simulink model "gg_plus_lc_platoon"  (R2019a)
settings: Solver=ode23t  StartTime=0.0  StopTime=70  FixedStep=0.1  MaxStep=0.01  RelTol=1e-3
InitFcn:
  | load vehStatesBus
libraries: simulink x120, powerlib_meascontrol x14, dspsigops x7, autolibshared x7
(part 4 of 7)

== system gg_plus_lc_platoon/Lo/Virtual Vehicle Following ==
  ego : Inport
  virtualLeader : Inport  Port=2
  leaderChange : Inport  Port=3
  extraSpaceFlag : Inport  Port=4
  Enable : EnablePort
  Bus Selector : BusSelector  OutputSignals=X,Xdot,u
  Bus Selector1 : BusSelector  OutputSignals=X,Xdot
  Chart : Stateflow chart  BlockKeywords=__PRM__SERIALIZED__DATA__:Stateflow Chart,Stateflow Diagram  TreatAsAtomicUnit=on
  Compare To Constant : simulink/Logic and Bit Operations/Compare To Constant  relop=>  const=0  OutDataTypeStr=boolean
  Compare To Constant1 : simulink/Logic and Bit Operations/Compare To Constant  relop=<  const=2*maxHeadwayError  OutDataTypeStr=boolean
  Compute Errors : Subsystem
  Mux : Mux  Inputs=2
  Scope : Scope  NumInputPorts=2
  Scope1 : Scope
  Sum : Sum  Inputs=-+|
  Sum6 : Sum  Inputs=|+-
  Terminator : Terminator
  Velocity Control Free Flow : Subsystem  TreatAsAtomicUnit=on
  Velocity Control Min : Subsystem  TreatAsAtomicUnit=on
  Virtual Leader Following : Subsystem  TreatAsAtomicUnit=on
  freeFlowVel : Constant  Value=freeFlowVel
  vMin : Constant  Value=vMin
  u : Outport  InitialOutput=0
  virtualErrors : Outport  Port=2  OutputWhenDisabled=reset  InitialOutput=[0, 0]
  virtualGap : Outport  Port=3  OutputWhenDisabled=reset  InitialOutput=[0]
  vLeaderInRange : Outport  Port=4
  wires:
  leaderChange/1 -> Virtual Leader Following/4(intReset), Compute Errors/6(velFilterReset)
  Compare To Constant1/1 -> Velocity Control Free Flow/3(intReset), vLeaderInRange/1, Chart/2(leaderWithinRange)
  Compare To Constant/1 -> Velocity Control Min/2(intReset)
  Velocity Control Free Flow/1(u) -> Chart/1(uFreeFlowVelControl)
  Sum/1 -> Velocity Control Min/1(ev), Chart/4(velDiff), Compare To Constant/1
  freeFlowVel/1 -> Sum6/1
  Chart/2(u) -> u/1, Scope/2
  Sum6/1 -> Velocity Control Free Flow/1(ev)
  virtualLeader/1 -> Bus Selector1/1
  Mux/1 -> virtualErrors/1
  vMin/1 -> Sum/2
  Compute Errors/1(eh) -> Compare To Constant1/1, Scope1/1, Virtual Leader Following/1(eh), Mux/1
  Bus Selector/3 -> Velocity Control Free Flow/2(realInput), Virtual Leader Following/3(realInput)  "<u>"
  ego/1 -> Bus Selector/1
  Virtual Leader Following/1(u) -> Chart/3(uVehFoll)  "uVehFoll"
  Bus Selector/2 -> Sum6/2, Sum/1, Compute Errors/2(vf)  "<Xdot>"
  Bus Selector/1 -> Compute Errors/1(xf)  "<X>"
  Compute Errors/3("gap ") -> virtualGap/1
  Compute Errors/4(unsafeFlag) -> Terminator/1
  Chart/1(state) -> Scope/1
  Bus Selector1/1 -> Compute Errors/3(xl)  "<X>"
  Velocity Control Min/1(u) -> Chart/5(uMinVelControl)  "uMinVelControl"
  Compute Errors/2(ev) -> Virtual Leader Following/2(ev), Mux/2
  extraSpaceFlag/1 -> Compute Errors/5(extraSpace)
  Bus Selector1/2 -> Compute Errors/4(vl)  "<Xdot>"

== system gg_plus_lc_platoon/Lo/controlChoice ==
  state : Inport
  follControl : Inport  Port=2
  leaderInRange : Inport  Port=3
  virtualFollControl : Inport  Port=4
  vLeaderInRange : Inport  Port=5
  ControlChoice : Stateflow chart  BlockKeywords=__PRM__SERIALIZED__DATA__:Stateflow Chart,Stateflow Diagram  TreatAsAtomicUnit=on
  Scope : Scope  NumInputPorts=2
  Scope1 : Scope  NumInputPorts=2
  u : Outport
  wires:
  state/1 -> Scope1/1, ControlChoice/1(state)
  leaderInRange/1 -> Scope1/2, ControlChoice/2(leaderInRange)
  virtualFollControl/1 -> Scope/2, ControlChoice/4(longAdjustmentData)
  follControl/1 -> Scope/1, ControlChoice/3(regVehFollData)
  ControlChoice/1(data) -> u/1  "u"
  vLeaderInRange/1 -> ControlChoice/5(vLeaderInRange)

== system gg_plus_lc_platoon/Lo/findLeader ==
  ego : Inport
  all : Inport  Port=2
  lcFlag : Inport  Port=3
  state : Inport  Port=4
  Compare To Constant : simulink/Logic and Bit Operations/Compare To Constant  relop=~=  const=4  OutDataTypeStr=boolean
  NOT : Logic  Operator=NOT  IconShape=distinctive  AllPortsSameDT=off  OutDataTypeStr=boolean
  OR : Logic  Operator=OR  IconShape=distinctive  AllPortsSameDT=off  OutDataTypeStr=boolean
  Selector : Selector  InputPortWidth=8  IndexOptions=Index vector (port)  Indices=[1]  OutputSizes=1
  Subsystem : Subsystem
  Vector Concatenate : Concatenate
  farAwayVeh : Subsystem
  leader : Outport
  leaderIdx : Outport  Port=2  InitialOutput=1
  wires:
  Vector Concatenate/1 -> Selector/1
  farAwayVeh/1(Out1) -> Vector Concatenate/2
  Selector/1 -> leader/1
  NOT/1 -> OR/1
  lcFlag/1 -> NOT/1
  OR/1 -> Subsystem/Enable
  Subsystem/1(idx) -> leaderIdx/1, Selector/2
  all/1 -> Subsystem/2(all), Vector Concatenate/1
  ego/1 -> Subsystem/1(ego), farAwayVeh/1(ego)
  state/1 -> Compare To Constant/1
  Compare To Constant/1 -> OR/2

== system gg_plus_lc_platoon/Lo/followerErrors ==
  ego : Inport
  follower : Inport  Port=2
  Bus Selector1 : BusSelector  OutputSignals=X,Xdot
  Bus Selector3 : BusSelector  OutputSignals=X,Xdot
  Mux : Mux  Inputs=2
  Sum3 : Sum  Inputs=-+|
  Terminator1 : Terminator
  gapToFollower : Subsystem
  errors : Outport
  wires:
  gapToFollower/2("gap ") -> Terminator1/1
  Sum3/1 -> Mux/2
  Bus Selector3/2 -> gapToFollower/2(vf), Sum3/1  "<Xdot>"
  follower/1 -> Bus Selector3/1
  gapToFollower/1(eh) -> Mux/1
  Bus Selector1/2 -> Sum3/2  "<Xdot>"
  Bus Selector3/1 -> gapToFollower/1(xf)  "<X>"
  ego/1 -> Bus Selector1/1
  Bus Selector1/1 -> gapToFollower/3(xl)  "<X>"
  Mux/1 -> errors/1

== system gg_plus_lc_platoon/Lo/maneuverState ==
  note: States are:
      | 0 - Lane keeping
      | 1 - Longitudinal Adjustment
      | 2 - Steady State
      | 3 - Safe to LC
      | 4 - Performing LC
      | 5 - LC is done
  longAdj : Inport
  steadyState : Inport  Port=2
  safeToVirtualFoll : Inport  Port=3
  canStartLC : Inport  Port=4
  lcDone : Inport  Port=5
  Enable : EnablePort
  AND{,1..3} (4 alike) : Logic  IconShape=distinctive  AllPortsSameDT=off  OutDataTypeStr=fixdt(1,16)
  Data Type Conversion : DataTypeConversion  OutMin=0  OutMax=1  OutDataTypeStr=fixdt(1,16)
  Scope : Scope  NumInputPorts=5
  Sum : Sum  Inputs=+++++
  state : Outport  InitialOutput=0
  wires:
  AND3/1 -> Scope/5, Sum/5
  AND2/1 -> AND3/1, Scope/4, Sum/4
  AND1/1 -> AND2/1, Scope/3, Sum/3
  AND/1 -> AND1/1, Scope/2, Sum/2
  Sum/1 -> state/1
  lcDone/1 -> AND3/2
  canStartLC/1 -> AND2/2
  safeToVirtualFoll/1 -> AND1/2
  steadyState/1 -> AND/2
  longAdj/1 -> Data Type Conversion/1, AND/1
  Data Type Conversion/1 -> Scope/1, Sum/1

== system gg_plus_lc_platoon/Lo/safeErrors ==
  errors : Inport
  AND : Logic  IconShape=distinctive  AllPortsSameDT=off  OutDataTypeStr=boolean
  Compare To Constant4 : simulink/Logic and Bit Operations/Compare To Constant  relop=>=  const=-0.1  OutDataTypeStr=boolean
  Demux : Demux  Outputs=2
  Demux1 : Demux  Outputs=2
  Memory : Memory
  Scope : Scope  NumInputPorts=2
  Triggered Subsystem1 : Subsystem  TreatAsAtomicUnit=on
  safetyFlag : Outport
  wires:
  Demux1/2 -> Scope/2
  Demux1/1 -> Scope/1
  Demux/2 -> AND/2
  Demux/1 -> AND/1
  AND/1 -> Triggered Subsystem1/Trigger
  errors/1 -> Compare To Constant4/1, Demux1/1
  Compare To Constant4/1 -> Demux/1
  Triggered Subsystem1/1(Out1) -> Memory/1
  Memory/1 -> safetyFlag/1

== system gg_plus_lc_platoon/Lo/virtualVehiclesManager ==
  all : Inport
  longAdj : Inport  Port=2
  lcFlag : Inport  Port=3
  lcDone : Inport  Port=4
  posInPlatoon : Inport  Port=5
  lcStrategy : Inport  Port=6
  Detect Change : simulink/Logic and Bit Operations/Detect Change  vinit=0  OutDataTypeStr=boolean
  MATLAB Function : MATLAB Function  TreatAsAtomicUnit=on
  MATLAB Function1 : MATLAB Function  TreatAsAtomicUnit=on
  Selector : Selector  InputPortWidth=7  IndexOptions=Index vector (port)  Indices=[1]  OutputSizes=1
  Selector1 : Selector  InputPortWidth=7  IndexOptions=Index vector (port)  Indices=[1]  OutputSizes=1
  Width : Width
  virtualVehs : Scope  NumInputPorts=2
  virtualLeader : Outport
  leaderChange : Outport  Port=2
  virtualFollower : Outport  Port=3
  wires:
  Detect Change/1 -> leaderChange/1
  Selector/1 -> virtualLeader/1
  all/1 -> Width/1, Selector1/1, Selector/1
  lcStrategy/1 -> MATLAB Function1/5(lcStrategy), MATLAB Function/6(lcStrategy)
  posInPlatoon/1 -> MATLAB Function1/4(posInPlatoon), MATLAB Function/5(posInPlatoon)
  lcFlag/1 -> MATLAB Function1/3(lcFlag), MATLAB Function/3(lcFlag)
  Width/1 -> MATLAB Function1/1(nVehicles), MATLAB Function/1(nVehicles)
  lcDone/1 -> MATLAB Function/4(lcDone)
  Selector1/1 -> virtualFollower/1
  longAdj/1 -> MATLAB Function1/2(longAdj), MATLAB Function/2(longAdj)
  MATLAB Function/1(virtualLeaderIdx) -> virtualVehs/1, Detect Change/1, Selector/2
  MATLAB Function1/1(virtualFollowerIdx) -> Selector1/2, virtualVehs/2

== system gg_plus_lc_platoon/p1/Lateral Control ==
  <Y> : Inport
  <r> : Inport  Port=2
  startLaneChange : Inport  Port=3
  yRef : Inport  Port=4
  Demux2 : Demux
  Full State Observer : Subsystem
  Gain1 : Gain  Gain=Klat  Multiplication=Matrix(K*u)
  Integrator : Integrator  InitialCondition=y0
  Mux : Mux  Inputs=2
  Pad : dspsigops/Pad  padAlong=Columns  dimsToPad=1  valSrc=Specify via dialog  padVal=0  spec=Output size  padNumOutRowsSpecMethod=User-specified  numOutRows=4  padNumOutColsSpecMethod=User-specified  numOutCols=1  isVarDimsMode=off  padBeginning=0  padEnd=0  outSizeMode=User-specified  outSize=1  padSigAt=End  trunc_flag=None  roundingMode=Floor  overflowMode=off  truncOrWrapMode=Truncate  wrap_flag=None
      settings: SourceProductName=DSP System Toolbox  SourceProductBaseCode=DS
  Rate Limiter : RateLimiter  RisingSlewLimit=maxDeltaDot  FallingSlewLimit=-maxDeltaDot  SampleTimeMode=inherited
  Saturation : Saturate  UpperLimit=maxDelta  LowerLimit=-maxDelta
  Scope : Scope  NumInputPorts=4
  Scope1 : Scope
  Sum : Sum  Inputs=|+-
  Sum2 : Sum  Inputs=|+-
  Triggered Subsystem1 : Subsystem  TreatAsAtomicUnit=on
  delta : Outport
  wires:
  yRef/1 -> Triggered Subsystem1/1(In1)
  startLaneChange/1 -> Triggered Subsystem1/Trigger
  <Y>/1 -> Mux/1
  Triggered Subsystem1/1(Out1) -> Sum2/1
  Demux2/3 -> Scope/3
  Saturation/1 -> Rate Limiter/1
  Sum2/1 -> Integrator/1
  Demux2/2 -> Scope/2
  Demux2/4 -> Scope/4
  Mux/1 -> Full State Observer/1(measuredOutputs)
  Pad/1 -> Sum/1
  Sum/1 -> Gain1/1
  Full State Observer/1(xhat) -> Demux2/1, Sum/2  "estStates"
  <r>/1 -> Mux/2
  Gain1/1 -> Saturation/1
  Integrator/1 -> Pad/1, Sum2/2
  Demux2/1 -> Scope/1
  Rate Limiter/1 -> delta/1, Scope1/1, Full State Observer/2(delta)  "delta"

== system gg_plus_lc_platoon/p1/Regular Vehicle Following ==
  ego : Inport
  leader : Inport  Port=2
  leaderChange : Inport  Port=3
  extraSpaceFlag : Inport  Port=4
  Bus Selector : BusSelector  OutputSignals=X,Xdot,u
  Bus Selector1 : BusSelector  OutputSignals=X,Xdot
  Compare To Constant : simulink/Logic and Bit Operations/Compare To Constant  relop=<  const=5*maxHeadwayError  OutDataTypeStr=boolean
  Compute Errors : Subsystem
  Constant : Constant  Value=0
  Mux : Mux  Inputs=2
  Rate Limiter : RateLimiter  RisingSlewLimit=maxJerk  FallingSlewLimit=minJerk  SampleTimeMode=inherited
  Rate Limiter1 : RateLimiter  RisingSlewLimit=maxComfJerk  FallingSlewLimit=minComfJerk  SampleTimeMode=inherited
  Scope : Scope
  Scope2 : Scope
  Switch : Switch  Criteria=u2 > Threshold
  Switch1 : Switch  Criteria=u2 > Threshold
  Veh Following : Subsystem  TreatAsAtomicUnit=on
  Velocity Control : Subsystem  TreatAsAtomicUnit=on
  XOR : Logic  Operator=XOR  IconShape=distinctive  AllPortsSameDT=off  OutDataTypeStr=boolean
  comf saturation : Saturate  UpperLimit=maxComfAccel  LowerLimit=minComfAccel
  eh : Scope
  output : Scope
  safe saturation : Saturate  UpperLimit=maxAcceleration  LowerLimit=minAcceleration
  veh foll state : Scope  NumInputPorts=2
  u : Outport
  errors : Outport  Port=2
  gap : Outport  Port=3
  leaderInRange : Outport  Port=4
  wires:
  Constant/1 -> Compute Errors/6(velFilterReset)
  XOR/1 -> Veh Following/4(intReset)
  Bus Selector1/2 -> Compute Errors/4(vl)  "<Xdot>"
  leader/1 -> Bus Selector1/1
  Compare To Constant/1 -> Velocity Control/3(intReset), XOR/2, leaderInRange/1, veh foll state/1, Switch/2
  Mux/1 -> errors/1
  Bus Selector1/1 -> Compute Errors/3(xl)  "<X>"
  Velocity Control/1(u) -> Switch/3
  Compute Errors/2(ev) -> Veh Following/2(ev), Mux/2
  comf saturation/1 -> Rate Limiter1/1
  safe saturation/1 -> Rate Limiter/1
  Rate Limiter/1 -> Switch1/1  "sat(u)"
  Switch1/1 -> output/1, u/1
  Switch/1 -> comf saturation/1, veh foll state/2, safe saturation/1
  Bus Selector/3 -> Velocity Control/2(realInput), Veh Following/3(realInput)  "<u>"
  Rate Limiter1/1 -> Switch1/3  "sat(u)"
  Compute Errors/4(unsafeFlag) -> Scope2/1, Switch1/2
  Compute Errors/3("gap ") -> gap/1
  ego/1 -> Bus Selector/1
  Compute Errors/1(eh) -> Mux/1, Veh Following/1(eh), Scope/1, Compare To Constant/1, eh/1
  extraSpaceFlag/1 -> Compute Errors/5(extraSpaceFlag)
  Veh Following/1(u) -> Switch/1
  Bus Selector/1 -> Compute Errors/1(xf)  "<X>"
  Bus Selector/2 -> Compute Errors/2(vf), Velocity Control/1(velocity)  "<Xdot>"
  leaderChange/1 -> XOR/1

== system gg_plus_lc_platoon/p1/Subsystem ==
  u : Inport
  state : Inport  Port=2
  Compare To Constant : simulink/Logic and Bit Operations/Compare To Constant  relop===  const=4  OutDataTypeStr=boolean
  Scope : Scope
  Switch1 : Switch  Criteria=u2 > Threshold
  comf saturation : Saturate  UpperLimit=maxComfAccel  LowerLimit=minComfAccel
  comf jerk : RateLimiter  RisingSlewLimit=maxComfJerk  FallingSlewLimit=minComfJerk  SampleTimeMode=inherited
  safe saturation : Saturate  UpperLimit=maxAcceleration  LowerLimit=minAcceleration
  safe jerk : RateLimiter  RisingSlewLimit=maxJerk  FallingSlewLimit=minJerk  SampleTimeMode=inherited
  sat(u) : Outport
  wires:
  safe saturation/1 -> safe jerk/1
  safe jerk/1 -> Switch1/1
  comf saturation/1 -> comf jerk/1
  state/1 -> Compare To Constant/1
  u/1 -> comf saturation/1, safe saturation/1
  comf jerk/1 -> Switch1/3
  Switch1/1 -> Scope/1, sat(u)/1
  Compare To Constant/1 -> Switch1/2

== system gg_plus_lc_platoon/p1/Subsystem1 ==
  u : Inport
  errors : Inport  Port=2
  virtualErrors : Inport  Port=3
  extraSpaceFlag : Inport  Port=4
  AND1 : Logic  Inputs=4  IconShape=distinctive  AllPortsSameDT=off  OutDataTypeStr=boolean
  Memory : Memory
  Triggered Subsystem1 : Subsystem  TreatAsAtomicUnit=on
  safeErrors1 : Subsystem
  safeErrors2 : Subsystem
  steadyState : Subsystem
  longAdjDone : Outport
  wires:
  u/1 -> steadyState/1(u)
  safeErrors1/1(safetyFlag) -> AND1/2
  steadyState/1(ssFlag) -> AND1/1
  extraSpaceFlag/1 -> AND1/4
  virtualErrors/1 -> safeErrors2/1(errors)
  safeErrors2/1(safetyFlag) -> AND1/3
  AND1/1 -> Triggered Subsystem1/Trigger
  Triggered Subsystem1/1(Out1) -> Memory/1
  errors/1 -> safeErrors1/1(errors)
  Memory/1 -> longAdjDone/1

== system gg_plus_lc_platoon/p1/Subsystem2 ==
  posInPlatoon : Inport
  strategy : Inport  Port=2
  platoonState : Inport  Port=3
  Enable : EnablePort
  MATLAB Function : MATLAB Function  TreatAsAtomicUnit=on
  longAdj : Outport
  wires:
  MATLAB Function/1(longAdjFlag) -> longAdj/1
  platoonState/1 -> MATLAB Function/3(platoonState)
  posInPlatoon/1 -> MATLAB Function/2(posInPlatoon)
  strategy/1 -> MATLAB Function/1(strategy)

== system gg_plus_lc_platoon/p1/Subsystem3 ==
  strategy : Inport
  platoonStates : Inport  Port=2
  Compare To Constant : simulink/Logic and Bit Operations/Compare To Constant  relop=>  const=1  OutDataTypeStr=boolean
  Compare To Constant1 : simulink/Logic and Bit Operations/Compare To Constant  relop=>  const=2  OutDataTypeStr=boolean
  OR : Logic  Operator=OR  IconShape=distinctive  AllPortsSameDT=off  OutDataTypeStr=boolean
  Selector : Selector  IndexOptions=Index vector (port)  Indices=[1 3]  OutputSizes=1
  Width : Width
  Out1 : Outport
  wires:
  Compare To Constant1/1 -> OR/2
  Selector/1 -> Compare To Constant1/1
  Width/1 -> Selector/2
  platoonStates/1 -> Selector/1, Width/1
  OR/1 -> Out1/1
  Compare To Constant/1 -> OR/1
  strategy/1 -> Compare To Constant/1

== system gg_plus_lc_platoon/p1/Triggered Subsystem ==
  Trigger : TriggerPort  VariantControl=Variant
  Constant : Constant
  lcFlag : Outport  InitialOutput=0
  wires:
  Constant/1 -> lcFlag/1

== system gg_plus_lc_platoon/p1/Virtual Vehicle Following ==
  ego : Inport
  virtualLeader : Inport  Port=2
  leaderChange : Inport  Port=3
  extraSpaceFlag : Inport  Port=4
  Enable : EnablePort
  Bus Selector : BusSelector  OutputSignals=X,Xdot,u
  Bus Selector1 : BusSelector  OutputSignals=X,Xdot
  Chart : Stateflow chart  BlockKeywords=__PRM__SERIALIZED__DATA__:Stateflow Chart,Stateflow Diagram  TreatAsAtomicUnit=on
  Compare To Constant : simulink/Logic and Bit Operations/Compare To Constant  relop=>  const=0  OutDataTypeStr=boolean
  Compare To Constant1 : simulink/Logic and Bit Operations/Compare To Constant  relop=<  const=2*maxHeadwayError  OutDataTypeStr=boolean
  Compute Errors : Subsystem
  Mux : Mux  Inputs=2
  Scope : Scope  NumInputPorts=2
  Scope1 : Scope
  Sum : Sum  Inputs=-+|
  Sum6 : Sum  Inputs=|+-
  Terminator : Terminator
  Velocity Control Free Flow : Subsystem  TreatAsAtomicUnit=on
  Velocity Control Min : Subsystem  TreatAsAtomicUnit=on
  Virtual Leader Following : Subsystem  TreatAsAtomicUnit=on
  freeFlowVel : Constant  Value=freeFlowVel
  vMin : Constant  Value=vMin
  u : Outport  InitialOutput=0
  virtualErrors : Outport  Port=2  OutputWhenDisabled=reset  InitialOutput=[0, 0]
  virtualGap : Outport  Port=3  OutputWhenDisabled=reset  InitialOutput=[0]
  vLeaderInRange : Outport  Port=4
  wires:
  Bus Selector1/2 -> Compute Errors/4(vl)  "<Xdot>"
  extraSpaceFlag/1 -> Compute Errors/5(extraSpace)
  Compute Errors/2(ev) -> Mux/2, Virtual Leader Following/2(ev)
  Velocity Control Min/1(u) -> Chart/5(uMinVelControl)  "uMinVelControl"
  Bus Selector1/1 -> Compute Errors/3(xl)  "<X>"
  Chart/1(state) -> Scope/1
  Compute Errors/4(unsafeFlag) -> Terminator/1
  Compute Errors/3("gap ") -> virtualGap/1
  Bus Selector/1 -> Compute Errors/1(xf)  "<X>"
  Bus Selector/2 -> Compute Errors/2(vf), Sum/1, Sum6/2  "<Xdot>"
  Virtual Leader Following/1(u) -> Chart/3(uVehFoll)  "uVehFoll"
  ego/1 -> Bus Selector/1
  Bus Selector/3 -> Virtual Leader Following/3(realInput), Velocity Control Free Flow/2(realInput)  "<u>"
  Compute Errors/1(eh) -> Mux/1, Virtual Leader Following/1(eh), Scope1/1, Compare To Constant1/1
  vMin/1 -> Sum/2
  Mux/1 -> virtualErrors/1
  virtualLeader/1 -> Bus Selector1/1
  Sum6/1 -> Velocity Control Free Flow/1(ev)
  Chart/2(u) -> Scope/2, u/1
  freeFlowVel/1 -> Sum6/1
  Sum/1 -> Compare To Constant/1, Chart/4(velDiff), Velocity Control Min/1(ev)
  Velocity Control Free Flow/1(u) -> Chart/1(uFreeFlowVelControl)
  Compare To Constant/1 -> Velocity Control Min/2(intReset)
  Compare To Constant1/1 -> Chart/2(leaderWithinRange), vLeaderInRange/1, Velocity Control Free Flow/3(intReset)
  leaderChange/1 -> Compute Errors/6(velFilterReset), Virtual Leader Following/4(intReset)

== system gg_plus_lc_platoon/p1/controlChoice ==
  state : Inport
  follControl : Inport  Port=2
  leaderInRange : Inport  Port=3
  virtualFollControl : Inport  Port=4
  vLeaderInRange : Inport  Port=5
  ControlChoice : Stateflow chart  BlockKeywords=__PRM__SERIALIZED__DATA__:Stateflow Chart,Stateflow Diagram  TreatAsAtomicUnit=on
  Scope : Scope  NumInputPorts=2
  Scope1 : Scope  NumInputPorts=2
  u : Outport
  wires:
  vLeaderInRange/1 -> ControlChoice/5(vLeaderInRange)
  ControlChoice/1(data) -> u/1  "u"
  follControl/1 -> ControlChoice/3(regVehFollData), Scope/1
  virtualFollControl/1 -> ControlChoice/4(longAdjustmentData), Scope/2
  leaderInRange/1 -> ControlChoice/2(leaderInRange), Scope1/2
  state/1 -> ControlChoice/1(state), Scope1/1

== system gg_plus_lc_platoon/p1/findLeader ==
  ego : Inport
  all : Inport  Port=2
  lcFlag : Inport  Port=3
  state : Inport  Port=4
  Compare To Constant : simulink/Logic and Bit Operations/Compare To Constant  relop=~=  const=4  OutDataTypeStr=boolean
  NOT : Logic  Operator=NOT  IconShape=distinctive  AllPortsSameDT=off  OutDataTypeStr=boolean
  OR : Logic  Operator=OR  IconShape=distinctive  AllPortsSameDT=off  OutDataTypeStr=boolean
  Selector : Selector  InputPortWidth=8  IndexOptions=Index vector (port)  Indices=[1]  OutputSizes=1
  Subsystem : Subsystem
  Vector Concatenate : Concatenate
  farAwayVeh : Subsystem
  leader : Outport
  leaderIdx : Outport  Port=2  InitialOutput=1
  wires:
  Compare To Constant/1 -> OR/2
  state/1 -> Compare To Constant/1
  ego/1 -> farAwayVeh/1(ego), Subsystem/1(ego)
  all/1 -> Vector Concatenate/1, Subsystem/2(all)
  Subsystem/1(idx) -> Selector/2, leaderIdx/1
  OR/1 -> Subsystem/Enable
  lcFlag/1 -> NOT/1
  NOT/1 -> OR/1
  Selector/1 -> leader/1
  farAwayVeh/1(Out1) -> Vector Concatenate/2
  Vector Concatenate/1 -> Selector/1

== system gg_plus_lc_platoon/p1/followerErrors ==
  ego : Inport
  follower : Inport  Port=2
  Bus Selector1 : BusSelector  OutputSignals=X,Xdot
  Bus Selector3 : BusSelector  OutputSignals=X,Xdot
  Mux : Mux  Inputs=2
  Sum3 : Sum  Inputs=-+|
  Terminator1 : Terminator
  gapToFollower : Subsystem
  errors : Outport
  wires:
  Mux/1 -> errors/1
  Bus Selector1/1 -> gapToFollower/3(xl)  "<X>"
  ego/1 -> Bus Selector1/1
  Bus Selector3/1 -> gapToFollower/1(xf)  "<X>"
  Bus Selector1/2 -> Sum3/2  "<Xdot>"
  gapToFollower/1(eh) -> Mux/1
  follower/1 -> Bus Selector3/1
  Bus Selector3/2 -> Sum3/1, gapToFollower/2(vf)  "<Xdot>"
  Sum3/1 -> Mux/2
  gapToFollower/2("gap ") -> Terminator1/1

== system gg_plus_lc_platoon/p1/maneuverState ==
  note: States are:
      | 0 - Lane keeping
      | 1 - Longitudinal Adjustment
      | 2 - Steady State
      | 3 - Safe to LC
      | 4 - Performing LC
      | 5 - LC is done
  longAdj : Inport
  steadyState : Inport  Port=2
  safeToVirtualFoll : Inport  Port=3
  canStartLC : Inport  Port=4
  lcDone : Inport  Port=5
  Enable : EnablePort
  AND{,1..3} (4 alike) : Logic  IconShape=distinctive  AllPortsSameDT=off  OutDataTypeStr=fixdt(1,16)
  Data Type Conversion : DataTypeConversion  OutMin=0  OutMax=1  OutDataTypeStr=fixdt(1,16)
  Scope : Scope  NumInputPorts=5
  Sum : Sum  Inputs=+++++
  state : Outport  InitialOutput=0
  wires:
  Data Type Conversion/1 -> Sum/1, Scope/1
  longAdj/1 -> AND/1, Data Type Conversion/1
  steadyState/1 -> AND/2
  safeToVirtualFoll/1 -> AND1/2
  canStartLC/1 -> AND2/2
  lcDone/1 -> AND3/2
  Sum/1 -> state/1
  AND/1 -> Sum/2, Scope/2, AND1/1
  AND1/1 -> Sum/3, Scope/3, AND2/1
  AND2/1 -> Sum/4, Scope/4, AND3/1
  AND3/1 -> Sum/5, Scope/5

== system gg_plus_lc_platoon/p1/safeErrors ==
  errors : Inport
  AND : Logic  IconShape=distinctive  AllPortsSameDT=off  OutDataTypeStr=boolean
  Compare To Constant4 : simulink/Logic and Bit Operations/Compare To Constant  relop=>=  const=-0.1  OutDataTypeStr=boolean
  Demux : Demux  Outputs=2
  Demux1 : Demux  Outputs=2
  Memory : Memory
  Scope : Scope  NumInputPorts=2
  Triggered Subsystem1 : Subsystem  TreatAsAtomicUnit=on
  safetyFlag : Outport
  wires:
  Memory/1 -> safetyFlag/1
  Triggered Subsystem1/1(Out1) -> Memory/1
  Compare To Constant4/1 -> Demux/1
  errors/1 -> Demux1/1, Compare To Constant4/1
  AND/1 -> Triggered Subsystem1/Trigger
  Demux/1 -> AND/1
  Demux/2 -> AND/2
  Demux1/1 -> Scope/1
  Demux1/2 -> Scope/2

== system gg_plus_lc_platoon/p1/virtualVehiclesManager ==
  all : Inport
  longAdj : Inport  Port=2
  lcFlag : Inport  Port=3
  lcDone : Inport  Port=4
  posInPlatoon : Inport  Port=5
  lcStrategy : Inport  Port=6
  Detect Change : simulink/Logic and Bit Operations/Detect Change  vinit=0  OutDataTypeStr=boolean
  MATLAB Function : MATLAB Function  TreatAsAtomicUnit=on
  MATLAB Function1 : MATLAB Function  TreatAsAtomicUnit=on
  Selector : Selector  InputPortWidth=7  IndexOptions=Index vector (port)  Indices=[1]  OutputSizes=1
  Selector1 : Selector  InputPortWidth=7  IndexOptions=Index vector (port)  Indices=[1]  OutputSizes=1
  Width : Width
  virtualVehs : Scope  NumInputPorts=2
  virtualLeader : Outport
  leaderChange : Outport  Port=2
  virtualFollower : Outport  Port=3
  wires:
  MATLAB Function1/1(virtualFollowerIdx) -> virtualVehs/2, Selector1/2
  MATLAB Function/1(virtualLeaderIdx) -> Selector/2, Detect Change/1, virtualVehs/1
  longAdj/1 -> MATLAB Function/2(longAdj), MATLAB Function1/2(longAdj)
  Selector1/1 -> virtualFollower/1
  lcDone/1 -> MATLAB Function/4(lcDone)
  Width/1 -> MATLAB Function/1(nVehicles), MATLAB Function1/1(nVehicles)
  lcFlag/1 -> MATLAB Function/3(lcFlag), MATLAB Function1/3(lcFlag)
  posInPlatoon/1 -> MATLAB Function/5(posInPlatoon), MATLAB Function1/4(posInPlatoon)
  lcStrategy/1 -> MATLAB Function/6(lcStrategy), MATLAB Function1/5(lcStrategy)
  all/1 -> Selector/1, Selector1/1, Width/1
  Selector/1 -> virtualLeader/1
  Detect Change/1 -> leaderChange/1

== system gg_plus_lc_platoon/p2/Lateral Control ==
  <Y> : Inport
  <r> : Inport  Port=2
  startLaneChange : Inport  Port=3
  yRef : Inport  Port=4
  Demux2 : Demux
  Full State Observer : Subsystem
  Gain1 : Gain  Gain=Klat  Multiplication=Matrix(K*u)
  Integrator : Integrator  InitialCondition=y0
  Mux : Mux  Inputs=2
  Pad : dspsigops/Pad  padAlong=Columns  dimsToPad=1  valSrc=Specify via dialog  padVal=0  spec=Output size  padNumOutRowsSpecMethod=User-specified  numOutRows=4  padNumOutColsSpecMethod=User-specified  numOutCols=1  isVarDimsMode=off  padBeginning=0  padEnd=0  outSizeMode=User-specified  outSize=1  padSigAt=End  trunc_flag=None  roundingMode=Floor  overflowMode=off  truncOrWrapMode=Truncate  wrap_flag=None
      settings: SourceProductName=DSP System Toolbox  SourceProductBaseCode=DS
  Rate Limiter : RateLimiter  RisingSlewLimit=maxDeltaDot  FallingSlewLimit=-maxDeltaDot  SampleTimeMode=inherited
  Saturation : Saturate  UpperLimit=maxDelta  LowerLimit=-maxDelta
  Scope : Scope  NumInputPorts=4
  Scope1 : Scope
  Sum : Sum  Inputs=|+-
  Sum2 : Sum  Inputs=|+-
  Triggered Subsystem1 : Subsystem  TreatAsAtomicUnit=on
  delta : Outport
  wires:
  Rate Limiter/1 -> Full State Observer/2(delta), Scope1/1, delta/1  "delta"
  Demux2/1 -> Scope/1
  Integrator/1 -> Sum2/2, Pad/1
  Gain1/1 -> Saturation/1
  <r>/1 -> Mux/2
  Full State Observer/1(xhat) -> Sum/2, Demux2/1  "estStates"
  Sum/1 -> Gain1/1
  Pad/1 -> Sum/1
  Mux/1 -> Full State Observer/1(measuredOutputs)
  Demux2/4 -> Scope/4
  Demux2/2 -> Scope/2
  Sum2/1 -> Integrator/1
  Saturation/1 -> Rate Limiter/1
  Demux2/3 -> Scope/3
  Triggered Subsystem1/1(Out1) -> Sum2/1
  <Y>/1 -> Mux/1
  startLaneChange/1 -> Triggered Subsystem1/Trigger
  yRef/1 -> Triggered Subsystem1/1(In1)

== system gg_plus_lc_platoon/p2/Regular Vehicle Following ==
  ego : Inport
  leader : Inport  Port=2
  leaderChange : Inport  Port=3
  extraSpaceFlag : Inport  Port=4
  Bus Selector : BusSelector  OutputSignals=X,Xdot,u
  Bus Selector1 : BusSelector  OutputSignals=X,Xdot
  Compare To Constant : simulink/Logic and Bit Operations/Compare To Constant  relop=<  const=5*maxHeadwayError  OutDataTypeStr=boolean
  Compute Errors : Subsystem
  Constant : Constant  Value=0
  Mux : Mux  Inputs=2
  Rate Limiter : RateLimiter  RisingSlewLimit=maxJerk  FallingSlewLimit=minJerk  SampleTimeMode=inherited
  Rate Limiter1 : RateLimiter  RisingSlewLimit=maxComfJerk  FallingSlewLimit=minComfJerk  SampleTimeMode=inherited
  Scope : Scope
  Scope2 : Scope
  Switch : Switch  Criteria=u2 > Threshold
  Switch1 : Switch  Criteria=u2 > Threshold
  Veh Following : Subsystem  TreatAsAtomicUnit=on
  Velocity Control : Subsystem  TreatAsAtomicUnit=on
  XOR : Logic  Operator=XOR  IconShape=distinctive  AllPortsSameDT=off  OutDataTypeStr=boolean
  comf saturation : Saturate  UpperLimit=maxComfAccel  LowerLimit=minComfAccel
  eh : Scope
  output : Scope
  safe saturation : Saturate  UpperLimit=maxAcceleration  LowerLimit=minAcceleration
  veh foll state : Scope  NumInputPorts=2
  u : Outport
  errors : Outport  Port=2
  gap : Outport  Port=3
  leaderInRange : Outport  Port=4
  wires:
  leaderChange/1 -> XOR/1
  Bus Selector/2 -> Velocity Control/1(velocity), Compute Errors/2(vf)  "<Xdot>"
  Bus Selector/1 -> Compute Errors/1(xf)  "<X>"
  Veh Following/1(u) -> Switch/1
  extraSpaceFlag/1 -> Compute Errors/5(extraSpaceFlag)
  Compute Errors/1(eh) -> eh/1, Compare To Constant/1, Scope/1, Veh Following/1(eh), Mux/1
  ego/1 -> Bus Selector/1
  Compute Errors/3("gap ") -> gap/1
  Compute Errors/4(unsafeFlag) -> Switch1/2, Scope2/1
  Rate Limiter1/1 -> Switch1/3  "sat(u)"
  Bus Selector/3 -> Veh Following/3(realInput), Velocity Control/2(realInput)  "<u>"
  Switch/1 -> safe saturation/1, veh foll state/2, comf saturation/1
  Switch1/1 -> u/1, output/1
  Rate Limiter/1 -> Switch1/1  "sat(u)"
  safe saturation/1 -> Rate Limiter/1
  comf saturation/1 -> Rate Limiter1/1
  Compute Errors/2(ev) -> Mux/2, Veh Following/2(ev)
  Velocity Control/1(u) -> Switch/3
  Bus Selector1/1 -> Compute Errors/3(xl)  "<X>"
  Mux/1 -> errors/1
  Compare To Constant/1 -> Switch/2, veh foll state/1, leaderInRange/1, XOR/2, Velocity Control/3(intReset)
  leader/1 -> Bus Selector1/1
  Bus Selector1/2 -> Compute Errors/4(vl)  "<Xdot>"
  XOR/1 -> Veh Following/4(intReset)
  Constant/1 -> Compute Errors/6(velFilterReset)

== system gg_plus_lc_platoon/p2/Subsystem ==
  u : Inport
  state : Inport  Port=2
  Compare To Constant : simulink/Logic and Bit Operations/Compare To Constant  relop===  const=4  OutDataTypeStr=boolean
  Scope : Scope
  Switch1 : Switch  Criteria=u2 > Threshold
  comf saturation : Saturate  UpperLimit=maxComfAccel  LowerLimit=minComfAccel
  comf jerk : RateLimiter  RisingSlewLimit=maxComfJerk  FallingSlewLimit=minComfJerk  SampleTimeMode=inherited
  safe saturation : Saturate  UpperLimit=maxAcceleration  LowerLimit=minAcceleration
  safe jerk : RateLimiter  RisingSlewLimit=maxJerk  FallingSlewLimit=minJerk  SampleTimeMode=inherited
  sat(u) : Outport
  wires:
  Compare To Constant/1 -> Switch1/2
  Switch1/1 -> sat(u)/1, Scope/1
  comf jerk/1 -> Switch1/3
  u/1 -> safe saturation/1, comf saturation/1
  state/1 -> Compare To Constant/1
  comf saturation/1 -> comf jerk/1
  safe jerk/1 -> Switch1/1
  safe saturation/1 -> safe jerk/1

== system gg_plus_lc_platoon/p2/Subsystem1 ==
  u : Inport
  errors : Inport  Port=2
  virtualErrors : Inport  Port=3
  extraSpaceFlag : Inport  Port=4
  AND1 : Logic  Inputs=4  IconShape=distinctive  AllPortsSameDT=off  OutDataTypeStr=boolean
  Memory : Memory
  Triggered Subsystem1 : Subsystem  TreatAsAtomicUnit=on
  safeErrors1 : Subsystem
  safeErrors2 : Subsystem
  steadyState : Subsystem
  longAdjDone : Outport
  wires:
  Memory/1 -> longAdjDone/1
  errors/1 -> safeErrors1/1(errors)
  Triggered Subsystem1/1(Out1) -> Memory/1
  AND1/1 -> Triggered Subsystem1/Trigger
  safeErrors2/1(safetyFlag) -> AND1/3
  virtualErrors/1 -> safeErrors2/1(errors)
  extraSpaceFlag/1 -> AND1/4
  steadyState/1(ssFlag) -> AND1/1
  safeErrors1/1(safetyFlag) -> AND1/2
  u/1 -> steadyState/1(u)

== system gg_plus_lc_platoon/p2/Subsystem2 ==
  posInPlatoon : Inport
  strategy : Inport  Port=2
  platoonState : Inport  Port=3
  Enable : EnablePort
  MATLAB Function : MATLAB Function  TreatAsAtomicUnit=on
  longAdj : Outport
  wires:
  strategy/1 -> MATLAB Function/1(strategy)
  posInPlatoon/1 -> MATLAB Function/2(posInPlatoon)
  platoonState/1 -> MATLAB Function/3(platoonState)
  MATLAB Function/1(longAdjFlag) -> longAdj/1

== system gg_plus_lc_platoon/p2/Subsystem3 ==
  strategy : Inport
  platoonStates : Inport  Port=2
  Compare To Constant : simulink/Logic and Bit Operations/Compare To Constant  relop=>  const=1  OutDataTypeStr=boolean
  Compare To Constant1 : simulink/Logic and Bit Operations/Compare To Constant  relop=>  const=2  OutDataTypeStr=boolean
  OR : Logic  Operator=OR  IconShape=distinctive  AllPortsSameDT=off  OutDataTypeStr=boolean
  Selector : Selector  IndexOptions=Index vector (port)  Indices=[1 3]  OutputSizes=1
  Width : Width
  Out1 : Outport
  wires:
  strategy/1 -> Compare To Constant/1
  Compare To Constant/1 -> OR/1
  OR/1 -> Out1/1
  platoonStates/1 -> Width/1, Selector/1
  Width/1 -> Selector/2
  Selector/1 -> Compare To Constant1/1
  Compare To Constant1/1 -> OR/2

== system gg_plus_lc_platoon/p2/Triggered Subsystem ==
  Trigger : TriggerPort  VariantControl=Variant
  Constant : Constant
  lcFlag : Outport  InitialOutput=0
  wires:
  Constant/1 -> lcFlag/1

== system gg_plus_lc_platoon/p2/Virtual Vehicle Following ==
  ego : Inport
  virtualLeader : Inport  Port=2
  leaderChange : Inport  Port=3
  extraSpaceFlag : Inport  Port=4
  Enable : EnablePort
  Bus Selector : BusSelector  OutputSignals=X,Xdot,u
  Bus Selector1 : BusSelector  OutputSignals=X,Xdot
  Chart : Stateflow chart  BlockKeywords=__PRM__SERIALIZED__DATA__:Stateflow Chart,Stateflow Diagram  TreatAsAtomicUnit=on
  Compare To Constant : simulink/Logic and Bit Operations/Compare To Constant  relop=>  const=0  OutDataTypeStr=boolean
  Compare To Constant1 : simulink/Logic and Bit Operations/Compare To Constant  relop=<  const=2*maxHeadwayError  OutDataTypeStr=boolean
  Compute Errors : Subsystem
  Mux : Mux  Inputs=2
  Scope : Scope  NumInputPorts=2
  Scope1 : Scope
  Sum : Sum  Inputs=-+|
  Sum6 : Sum  Inputs=|+-
  Terminator : Terminator
  Velocity Control Free Flow : Subsystem  TreatAsAtomicUnit=on
  Velocity Control Min : Subsystem  TreatAsAtomicUnit=on
  Virtual Leader Following : Subsystem  TreatAsAtomicUnit=on
  freeFlowVel : Constant  Value=freeFlowVel
  vMin : Constant  Value=vMin
  u : Outport  InitialOutput=0
  virtualErrors : Outport  Port=2  OutputWhenDisabled=reset  InitialOutput=[0, 0]
  virtualGap : Outport  Port=3  OutputWhenDisabled=reset  InitialOutput=[0]
  vLeaderInRange : Outport  Port=4
  wires:
  leaderChange/1 -> Virtual Leader Following/4(intReset), Compute Errors/6(velFilterReset)
  Compare To Constant1/1 -> Velocity Control Free Flow/3(intReset), vLeaderInRange/1, Chart/2(leaderWithinRange)
  Compare To Constant/1 -> Velocity Control Min/2(intReset)
  Velocity Control Free Flow/1(u) -> Chart/1(uFreeFlowVelControl)
  Sum/1 -> Velocity Control Min/1(ev), Chart/4(velDiff), Compare To Constant/1
  freeFlowVel/1 -> Sum6/1
  Chart/2(u) -> u/1, Scope/2
  Sum6/1 -> Velocity Control Free Flow/1(ev)
  virtualLeader/1 -> Bus Selector1/1
  Mux/1 -> virtualErrors/1
  vMin/1 -> Sum/2
  Compute Errors/1(eh) -> Compare To Constant1/1, Scope1/1, Virtual Leader Following/1(eh), Mux/1
  Bus Selector/3 -> Velocity Control Free Flow/2(realInput), Virtual Leader Following/3(realInput)  "<u>"
  ego/1 -> Bus Selector/1
  Virtual Leader Following/1(u) -> Chart/3(uVehFoll)  "uVehFoll"
  Bus Selector/2 -> Sum6/2, Sum/1, Compute Errors/2(vf)  "<Xdot>"
  Bus Selector/1 -> Compute Errors/1(xf)  "<X>"
  Compute Errors/3("gap ") -> virtualGap/1
  Compute Errors/4(unsafeFlag) -> Terminator/1
  Chart/1(state) -> Scope/1
  Bus Selector1/1 -> Compute Errors/3(xl)  "<X>"
  Velocity Control Min/1(u) -> Chart/5(uMinVelControl)  "uMinVelControl"
  Compute Errors/2(ev) -> Virtual Leader Following/2(ev), Mux/2
  extraSpaceFlag/1 -> Compute Errors/5(extraSpace)
  Bus Selector1/2 -> Compute Errors/4(vl)  "<Xdot>"

== system gg_plus_lc_platoon/p2/controlChoice ==
  state : Inport
  follControl : Inport  Port=2
  leaderInRange : Inport  Port=3
  virtualFollControl : Inport  Port=4
  vLeaderInRange : Inport  Port=5
  ControlChoice : Stateflow chart  BlockKeywords=__PRM__SERIALIZED__DATA__:Stateflow Chart,Stateflow Diagram  TreatAsAtomicUnit=on
  Scope : Scope  NumInputPorts=2
  Scope1 : Scope  NumInputPorts=2
  u : Outport
  wires:
  state/1 -> Scope1/1, ControlChoice/1(state)
  leaderInRange/1 -> Scope1/2, ControlChoice/2(leaderInRange)
  virtualFollControl/1 -> Scope/2, ControlChoice/4(longAdjustmentData)
  follControl/1 -> Scope/1, ControlChoice/3(regVehFollData)
  ControlChoice/1(data) -> u/1  "u"
  vLeaderInRange/1 -> ControlChoice/5(vLeaderInRange)

== system gg_plus_lc_platoon/p2/findLeader ==
  ego : Inport
  all : Inport  Port=2
  lcFlag : Inport  Port=3
  state : Inport  Port=4
  Compare To Constant : simulink/Logic and Bit Operations/Compare To Constant  relop=~=  const=4  OutDataTypeStr=boolean
  NOT : Logic  Operator=NOT  IconShape=distinctive  AllPortsSameDT=off  OutDataTypeStr=boolean
  OR : Logic  Operator=OR  IconShape=distinctive  AllPortsSameDT=off  OutDataTypeStr=boolean
  Selector : Selector  InputPortWidth=8  IndexOptions=Index vector (port)  Indices=[1]  OutputSizes=1
  Subsystem : Subsystem
  Vector Concatenate : Concatenate
  farAwayVeh : Subsystem
  leader : Outport
  leaderIdx : Outport  Port=2  InitialOutput=1
  wires:
  Vector Concatenate/1 -> Selector/1
  farAwayVeh/1(Out1) -> Vector Concatenate/2
  Selector/1 -> leader/1
  NOT/1 -> OR/1
  lcFlag/1 -> NOT/1
  OR/1 -> Subsystem/Enable
  Subsystem/1(idx) -> leaderIdx/1, Selector/2
  all/1 -> Subsystem/2(all), Vector Concatenate/1
  ego/1 -> Subsystem/1(ego), farAwayVeh/1(ego)
  state/1 -> Compare To Constant/1
  Compare To Constant/1 -> OR/2

== system gg_plus_lc_platoon/p2/followerErrors ==
  ego : Inport
  follower : Inport  Port=2
  Bus Selector1 : BusSelector  OutputSignals=X,Xdot
  Bus Selector3 : BusSelector  OutputSignals=X,Xdot
  Mux : Mux  Inputs=2
  Sum3 : Sum  Inputs=-+|
  Terminator1 : Terminator
  gapToFollower : Subsystem
  errors : Outport
  wires:
  gapToFollower/2("gap ") -> Terminator1/1
  Sum3/1 -> Mux/2
  Bus Selector3/2 -> gapToFollower/2(vf), Sum3/1  "<Xdot>"
  follower/1 -> Bus Selector3/1
  gapToFollower/1(eh) -> Mux/1
  Bus Selector1/2 -> Sum3/2  "<Xdot>"
  Bus Selector3/1 -> gapToFollower/1(xf)  "<X>"
  ego/1 -> Bus Selector1/1
  Bus Selector1/1 -> gapToFollower/3(xl)  "<X>"
  Mux/1 -> errors/1

== system gg_plus_lc_platoon/p2/maneuverState ==
  note: States are:
      | 0 - Lane keeping
      | 1 - Longitudinal Adjustment
      | 2 - Steady State
      | 3 - Safe to LC
      | 4 - Performing LC
      | 5 - LC is done
  longAdj : Inport
  steadyState : Inport  Port=2
  safeToVirtualFoll : Inport  Port=3
  canStartLC : Inport  Port=4
  lcDone : Inport  Port=5
  Enable : EnablePort
  AND{,1..3} (4 alike) : Logic  IconShape=distinctive  AllPortsSameDT=off  OutDataTypeStr=fixdt(1,16)
  Data Type Conversion : DataTypeConversion  OutMin=0  OutMax=1  OutDataTypeStr=fixdt(1,16)
  Scope : Scope  NumInputPorts=5
  Sum : Sum  Inputs=+++++
  state : Outport  InitialOutput=0
  wires:
  AND3/1 -> Scope/5, Sum/5
  AND2/1 -> AND3/1, Scope/4, Sum/4
  AND1/1 -> AND2/1, Scope/3, Sum/3
  AND/1 -> AND1/1, Scope/2, Sum/2
  Sum/1 -> state/1
  lcDone/1 -> AND3/2
  canStartLC/1 -> AND2/2
  safeToVirtualFoll/1 -> AND1/2
  steadyState/1 -> AND/2
  longAdj/1 -> Data Type Conversion/1, AND/1
  Data Type Conversion/1 -> Scope/1, Sum/1

== system gg_plus_lc_platoon/p2/safeErrors ==
  errors : Inport
  AND : Logic  IconShape=distinctive  AllPortsSameDT=off  OutDataTypeStr=boolean
  Compare To Constant4 : simulink/Logic and Bit Operations/Compare To Constant  relop=>=  const=-0.1  OutDataTypeStr=boolean
  Demux : Demux  Outputs=2
  Demux1 : Demux  Outputs=2
  Memory : Memory
  Scope : Scope  NumInputPorts=2
  Triggered Subsystem1 : Subsystem  TreatAsAtomicUnit=on
  safetyFlag : Outport
  wires:
  Demux1/2 -> Scope/2
  Demux1/1 -> Scope/1
  Demux/2 -> AND/2
  Demux/1 -> AND/1
  AND/1 -> Triggered Subsystem1/Trigger
  errors/1 -> Compare To Constant4/1, Demux1/1
  Compare To Constant4/1 -> Demux/1
  Triggered Subsystem1/1(Out1) -> Memory/1
  Memory/1 -> safetyFlag/1

== system gg_plus_lc_platoon/p2/virtualVehiclesManager ==
  all : Inport
  longAdj : Inport  Port=2
  lcFlag : Inport  Port=3
  lcDone : Inport  Port=4
  posInPlatoon : Inport  Port=5
  lcStrategy : Inport  Port=6
  Detect Change : simulink/Logic and Bit Operations/Detect Change  vinit=0  OutDataTypeStr=boolean
  MATLAB Function : MATLAB Function  TreatAsAtomicUnit=on
  MATLAB Function1 : MATLAB Function  TreatAsAtomicUnit=on
  Selector : Selector  InputPortWidth=7  IndexOptions=Index vector (port)  Indices=[1]  OutputSizes=1
  Selector1 : Selector  InputPortWidth=7  IndexOptions=Index vector (port)  Indices=[1]  OutputSizes=1
  Width : Width
  virtualVehs : Scope  NumInputPorts=2
  virtualLeader : Outport
  leaderChange : Outport  Port=2
  virtualFollower : Outport  Port=3
  wires:
  Detect Change/1 -> leaderChange/1
  Selector/1 -> virtualLeader/1
  all/1 -> Width/1, Selector1/1, Selector/1
  lcStrategy/1 -> MATLAB Function1/5(lcStrategy), MATLAB Function/6(lcStrategy)
  posInPlatoon/1 -> MATLAB Function1/4(posInPlatoon), MATLAB Function/5(posInPlatoon)
  lcFlag/1 -> MATLAB Function1/3(lcFlag), MATLAB Function/3(lcFlag)
  Width/1 -> MATLAB Function1/1(nVehicles), MATLAB Function/1(nVehicles)
  lcDone/1 -> MATLAB Function/4(lcDone)
  Selector1/1 -> virtualFollower/1
  longAdj/1 -> MATLAB Function1/2(longAdj), MATLAB Function/2(longAdj)
  MATLAB Function/1(virtualLeaderIdx) -> virtualVehs/1, Detect Change/1, Selector/2
  MATLAB Function1/1(virtualFollowerIdx) -> Selector1/2, virtualVehs/2

== system gg_plus_lc_platoon/p3/Lateral Control ==
  <Y> : Inport
  <r> : Inport  Port=2
  startLaneChange : Inport  Port=3
  yRef : Inport  Port=4
  Demux2 : Demux
  Full State Observer : Subsystem
  Gain1 : Gain  Gain=Klat  Multiplication=Matrix(K*u)
  Integrator : Integrator  InitialCondition=y0
  Mux : Mux  Inputs=2
  Pad : dspsigops/Pad  padAlong=Columns  dimsToPad=1  valSrc=Specify via dialog  padVal=0  spec=Output size  padNumOutRowsSpecMethod=User-specified  numOutRows=4  padNumOutColsSpecMethod=User-specified  numOutCols=1  isVarDimsMode=off  padBeginning=0  padEnd=0  outSizeMode=User-specified  outSize=1  padSigAt=End  trunc_flag=None  roundingMode=Floor  overflowMode=off  truncOrWrapMode=Truncate  wrap_flag=None
      settings: SourceProductName=DSP System Toolbox  SourceProductBaseCode=DS
  Rate Limiter : RateLimiter  RisingSlewLimit=maxDeltaDot  FallingSlewLimit=-maxDeltaDot  SampleTimeMode=inherited
  Saturation : Saturate  UpperLimit=maxDelta  LowerLimit=-maxDelta
  Scope : Scope  NumInputPorts=4
  Scope1 : Scope
  Sum : Sum  Inputs=|+-
  Sum2 : Sum  Inputs=|+-
  Triggered Subsystem1 : Subsystem  TreatAsAtomicUnit=on
  delta : Outport
  wires:
  Rate Limiter/1 -> Full State Observer/2(delta), Scope1/1, delta/1  "delta"
  Demux2/1 -> Scope/1
  Integrator/1 -> Sum2/2, Pad/1
  Gain1/1 -> Saturation/1
  <r>/1 -> Mux/2
  Full State Observer/1(xhat) -> Sum/2, Demux2/1  "estStates"
  Sum/1 -> Gain1/1
  Pad/1 -> Sum/1
  Mux/1 -> Full State Observer/1(measuredOutputs)
  Demux2/4 -> Scope/4
  Demux2/2 -> Scope/2
  Sum2/1 -> Integrator/1
  Saturation/1 -> Rate Limiter/1
  Demux2/3 -> Scope/3
  Triggered Subsystem1/1(Out1) -> Sum2/1
  <Y>/1 -> Mux/1
  startLaneChange/1 -> Triggered Subsystem1/Trigger
  yRef/1 -> Triggered Subsystem1/1(In1)

== system gg_plus_lc_platoon/p3/Regular Vehicle Following ==
  ego : Inport
  leader : Inport  Port=2
  leaderChange : Inport  Port=3
  extraSpaceFlag : Inport  Port=4
  Bus Selector : BusSelector  OutputSignals=X,Xdot,u
  Bus Selector1 : BusSelector  OutputSignals=X,Xdot
  Compare To Constant : simulink/Logic and Bit Operations/Compare To Constant  relop=<  const=5*maxHeadwayError  OutDataTypeStr=boolean
  Compute Errors : Subsystem
  Constant : Constant  Value=0
  Mux : Mux  Inputs=2
  Rate Limiter : RateLimiter  RisingSlewLimit=maxJerk  FallingSlewLimit=minJerk  SampleTimeMode=inherited
  Rate Limiter1 : RateLimiter  RisingSlewLimit=maxComfJerk  FallingSlewLimit=minComfJerk  SampleTimeMode=inherited
  Scope : Scope
  Scope2 : Scope
  Switch : Switch  Criteria=u2 > Threshold
  Switch1 : Switch  Criteria=u2 > Threshold
  Veh Following : Subsystem  TreatAsAtomicUnit=on
  Velocity Control : Subsystem  TreatAsAtomicUnit=on
  XOR : Logic  Operator=XOR  IconShape=distinctive  AllPortsSameDT=off  OutDataTypeStr=boolean
  comf saturation : Saturate  UpperLimit=maxComfAccel  LowerLimit=minComfAccel
  eh : Scope
  output : Scope
  safe saturation : Saturate  UpperLimit=maxAcceleration  LowerLimit=minAcceleration
  veh foll state : Scope  NumInputPorts=2
  u : Outport
  errors : Outport  Port=2
  gap : Outport  Port=3
  leaderInRange : Outport  Port=4
  wires:
  leaderChange/1 -> XOR/1
  Bus Selector/2 -> Velocity Control/1(velocity), Compute Errors/2(vf)  "<Xdot>"
  Bus Selector/1 -> Compute Errors/1(xf)  "<X>"
  Veh Following/1(u) -> Switch/1
  extraSpaceFlag/1 -> Compute Errors/5(extraSpaceFlag)
  Compute Errors/1(eh) -> eh/1, Compare To Constant/1, Scope/1, Veh Following/1(eh), Mux/1
  ego/1 -> Bus Selector/1
  Compute Errors/3("gap ") -> gap/1
  Compute Errors/4(unsafeFlag) -> Switch1/2, Scope2/1
  Rate Limiter1/1 -> Switch1/3  "sat(u)"
  Bus Selector/3 -> Veh Following/3(realInput), Velocity Control/2(realInput)  "<u>"
  Switch/1 -> safe saturation/1, veh foll state/2, comf saturation/1
  Switch1/1 -> u/1, output/1
  Rate Limiter/1 -> Switch1/1  "sat(u)"
  safe saturation/1 -> Rate Limiter/1
  comf saturation/1 -> Rate Limiter1/1
  Compute Errors/2(ev) -> Mux/2, Veh Following/2(ev)
  Velocity Control/1(u) -> Switch/3
  Bus Selector1/1 -> Compute Errors/3(xl)  "<X>"
  Mux/1 -> errors/1
  Compare To Constant/1 -> Switch/2, veh foll state/1, leaderInRange/1, XOR/2, Velocity Control/3(intReset)
  leader/1 -> Bus Selector1/1
  Bus Selector1/2 -> Compute Errors/4(vl)  "<Xdot>"
  XOR/1 -> Veh Following/4(intReset)
  Constant/1 -> Compute Errors/6(velFilterReset)

== system gg_plus_lc_platoon/p3/Subsystem ==
  u : Inport
  state : Inport  Port=2
  Compare To Constant : simulink/Logic and Bit Operations/Compare To Constant  relop===  const=4  OutDataTypeStr=boolean
  Scope : Scope
  Switch1 : Switch  Criteria=u2 > Threshold
  comf saturation : Saturate  UpperLimit=maxComfAccel  LowerLimit=minComfAccel
  comf jerk : RateLimiter  RisingSlewLimit=maxComfJerk  FallingSlewLimit=minComfJerk  SampleTimeMode=inherited
  safe saturation : Saturate  UpperLimit=maxAcceleration  LowerLimit=minAcceleration
  safe jerk : RateLimiter  RisingSlewLimit=maxJerk  FallingSlewLimit=minJerk  SampleTimeMode=inherited
  sat(u) : Outport
  wires:
  Compare To Constant/1 -> Switch1/2
  Switch1/1 -> sat(u)/1, Scope/1
  comf jerk/1 -> Switch1/3
  u/1 -> safe saturation/1, comf saturation/1
  state/1 -> Compare To Constant/1
  comf saturation/1 -> comf jerk/1
  safe jerk/1 -> Switch1/1
  safe saturation/1 -> safe jerk/1

== system gg_plus_lc_platoon/p3/Subsystem1 ==
  u : Inport
  errors : Inport  Port=2
  virtualErrors : Inport  Port=3
  extraSpaceFlag : Inport  Port=4
  AND1 : Logic  Inputs=4  IconShape=distinctive  AllPortsSameDT=off  OutDataTypeStr=boolean
  Memory : Memory
  Triggered Subsystem1 : Subsystem  TreatAsAtomicUnit=on
  safeErrors1 : Subsystem
  safeErrors2 : Subsystem
  steadyState : Subsystem
  longAdjDone : Outport
  wires:
  Memory/1 -> longAdjDone/1
  errors/1 -> safeErrors1/1(errors)
  Triggered Subsystem1/1(Out1) -> Memory/1
  AND1/1 -> Triggered Subsystem1/Trigger
  safeErrors2/1(safetyFlag) -> AND1/3
  virtualErrors/1 -> safeErrors2/1(errors)
  extraSpaceFlag/1 -> AND1/4
  steadyState/1(ssFlag) -> AND1/1
  safeErrors1/1(safetyFlag) -> AND1/2
  u/1 -> steadyState/1(u)

== system gg_plus_lc_platoon/p3/Subsystem2 ==
  posInPlatoon : Inport
  strategy : Inport  Port=2
  platoonState : Inport  Port=3
  Enable : EnablePort
  MATLAB Function : MATLAB Function  TreatAsAtomicUnit=on
  longAdj : Outport
  wires:
  strategy/1 -> MATLAB Function/1(strategy)
  posInPlatoon/1 -> MATLAB Function/2(posInPlatoon)
  platoonState/1 -> MATLAB Function/3(platoonState)
  MATLAB Function/1(longAdjFlag) -> longAdj/1

== system gg_plus_lc_platoon/p3/Subsystem3 ==
  strategy : Inport
  platoonStates : Inport  Port=2
  Compare To Constant : simulink/Logic and Bit Operations/Compare To Constant  relop=>  const=1  OutDataTypeStr=boolean
  Compare To Constant1 : simulink/Logic and Bit Operations/Compare To Constant  relop=>  const=2  OutDataTypeStr=boolean
  OR : Logic  Operator=OR  IconShape=distinctive  AllPortsSameDT=off  OutDataTypeStr=boolean
  Selector : Selector  IndexOptions=Index vector (port)  Indices=[1 3]  OutputSizes=1
  Width : Width
  Out1 : Outport
  wires:
  strategy/1 -> Compare To Constant/1
  Compare To Constant/1 -> OR/1
  OR/1 -> Out1/1
  platoonStates/1 -> Width/1, Selector/1
  Width/1 -> Selector/2
  Selector/1 -> Compare To Constant1/1
  Compare To Constant1/1 -> OR/2

== system gg_plus_lc_platoon/p3/Triggered Subsystem ==
  Trigger : TriggerPort  VariantControl=Variant
  Constant : Constant
  lcFlag : Outport  InitialOutput=0
  wires:
  Constant/1 -> lcFlag/1
